simulink model "Labhalleffect"  (R2026a)
settings: Solver=FixedStepDiscrete  StopTime=10  FixedStep=0.001
undefined symbols (not defined in the file or in its folder): Blocking, Non
libraries: amg_usbconverter_n_connect_lib x2
settings Model: Creator=pboon  LastModifiedBy=Admin

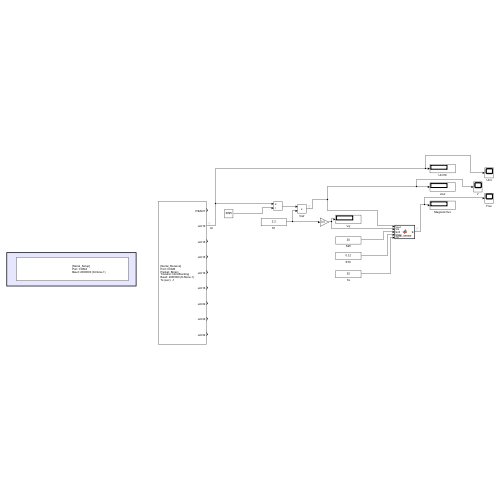
[thumbnail: Simulink's stored preview of the top-level diagram]
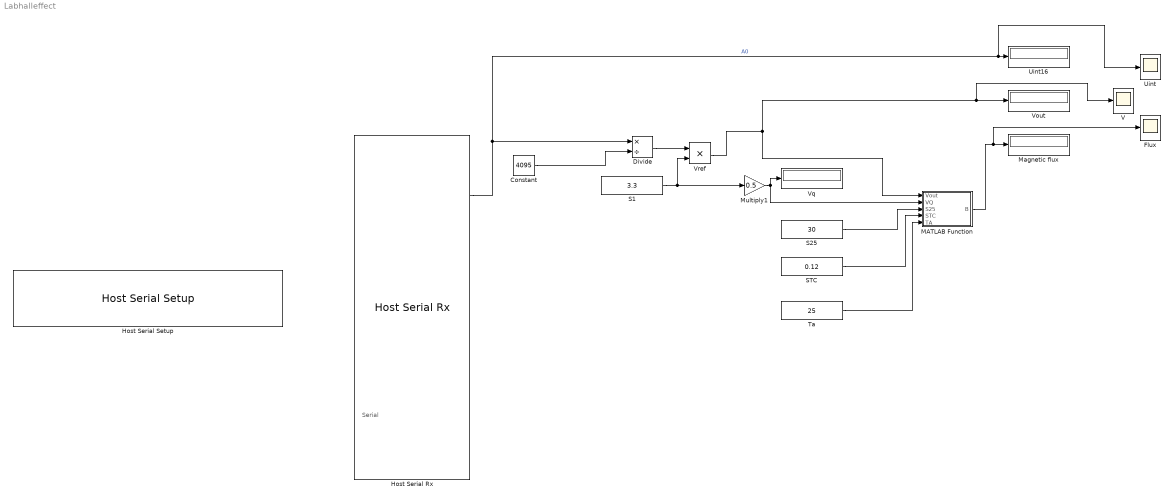
== system Labhalleffect ==
  note: Serial
  Constant : Constant  Value=4095
  Divide : Product  Inputs=*/
  Flux : Scope
      settings: ActiveDisplayYMinimum=-1.2984175919784593  ActiveDisplayYMaximum=3.1861276356275692
  Host Serial Rx : amg_usbconverter_n_connect_lib/Host Serial Rx  conf=rx  port=<auto>  baudrate=2000000  databits=8  parity=None  stopbit=1  flowcontrol=None  transfer=Non-Blocking  timeout=5  packetmode=Binary  enableinitialvalues=off  initialvalues=[]  binheader='25'  binterminator='4E 4E'  porttype_double=0  porttype_single=0  porttype_int8=0  porttype_uint8=0  porttype_int16=0  porttype_uint16=5  porttype_int32=0  porttype_uint32=3  asciiformat='%d,%f'  rx_asciiterminator="CRLF (0x0D 0x0A - \"\\r\\n\")"  tx_asciiterminator="CRLF (0x0D 0x0A - \"\\r\\n\")"  sampletime=0.001  enablecustomportlabel=off  cinputportlabel=0  coutputportlabel=A  portpinstr=0  blockid=HostSerialRx  inputporttype=[]  inputportwidth=[]  inputportlabel={}  outputporttype=[3 5 5 5 5 5 7 7 7]  outputportwidth=[1 1 1 1 1 1 1 1 1]  outputportlabel={'READY','uint16','uint16','uint16','uint16','uint16','uint32','uint32','uint32'}  compat=0  optionstring=[]  autoport='COM4'
  Host Serial Setup : amg_usbconverter_n_connect_lib/Host Serial Setup  conf=setup  port=<auto>  baudrate=2000000  databits=8  parity=None  stopbit=1  flowcontrol=None  transfer=Blocking  timeout=2  packetmode=Binary  initialvalues=[]  binheader='7E 7E'  binterminator='03 03'  porttype_double=0  porttype_single=1  porttype_int8=0  porttype_uint8=0  porttype_int16=0  porttype_uint16=0  porttype_int32=0  porttype_uint32=2  asciiformat='%d %u %x'  rx_asciiterminator="CRLF (0x0D 0x0A - \"\\r\\n\")"  tx_asciiterminator="CRLF (0x0D 0x0A - \"\\r\\n\")"  sampletime=-1  enablecustomportlabel=off  cinputportlabel=0  coutputportlabel=A  portpinstr=0  blockid=HostSerialSetup  inputporttype=[]  inputportwidth=[]  inputportlabel={}  outputporttype=[]  outputportwidth=[]  outputportlabel={}  compat=0  optionstring=[]  autoport='COM4'
  MATLAB Function : MATLAB Function  TreatAsAtomicUnit=on
  Magnetic flux : Display
  Multiply1 : Gain  Gain=0.5
  S1 : Constant  Value=3.3
  S25 : Constant  Value=30
  STC : Constant  Value=0.12
  Ta : Constant  Value=25
  Uint : Scope
      settings: ActiveDisplayYMinimum=1950.776416185875  ActiveDisplayYMaximum=2091.8745387233489
  Uint16 : Display
  V : Scope
      settings: ActiveDisplayYMinimum=1.6307600732600733  ActiveDisplayYMaximum=1.6660164835164837  DataLoggingVariableName=ScopeData3
  Vout : Display
  Vq : Display
  Vref : Product
  wires:
  Host Serial Rx/2 -> Divide/1, Uint/1, Uint16/1  "A0"
  Constant/1 -> Divide/2
  Divide/1 -> Vref/1
  Multiply1/1 -> Vq/1, MATLAB Function/2(VQ)
  S25/1 -> MATLAB Function/3(S25)
  STC/1 -> MATLAB Function/4(STC)
  Ta/1 -> MATLAB Function/5(TA)
  MATLAB Function/1(B) -> Flux/1, Magnetic flux/1
  S1/1 -> Multiply1/1, Vref/2
  Vref/1 -> MATLAB Function/1(Vout), V/1, Vout/1

== matlab function Labhalleffect/MATLAB Function ==
  data: Vout input; B output; VQ input; S25 input; STC input; TA input
function B = hall_sensor(Vout, VQ, S25, STC, TA)

B = (Vout - VQ) / (S25 * (1 + STC * (TA - 25)));
end
